simulink model "commit9"  (R2022a)
settings: Solver=VariableStepAuto  StartTime=0.0  StopTime=50  RelTol=1e-3
InitFcn:
  | uav_param, LQR_maker
undefined symbols (not defined in the file or in its folder): auto_LQR, Continuous, drawQuad, ff_splitter1, ff_splitter2, gr_eff, intrcptr_traj3, OL_LIN_maker, plotmavstatevariables, pos_comprtr, splitter1, Time, uav_P
libraries: ctrlSharedLib x1
settings Model: Creator=Abhi  LastModifiedBy=Abhi

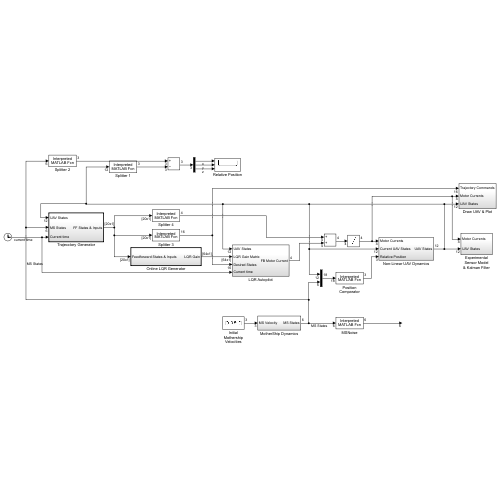
[thumbnail: Simulink's stored preview of the top-level diagram]
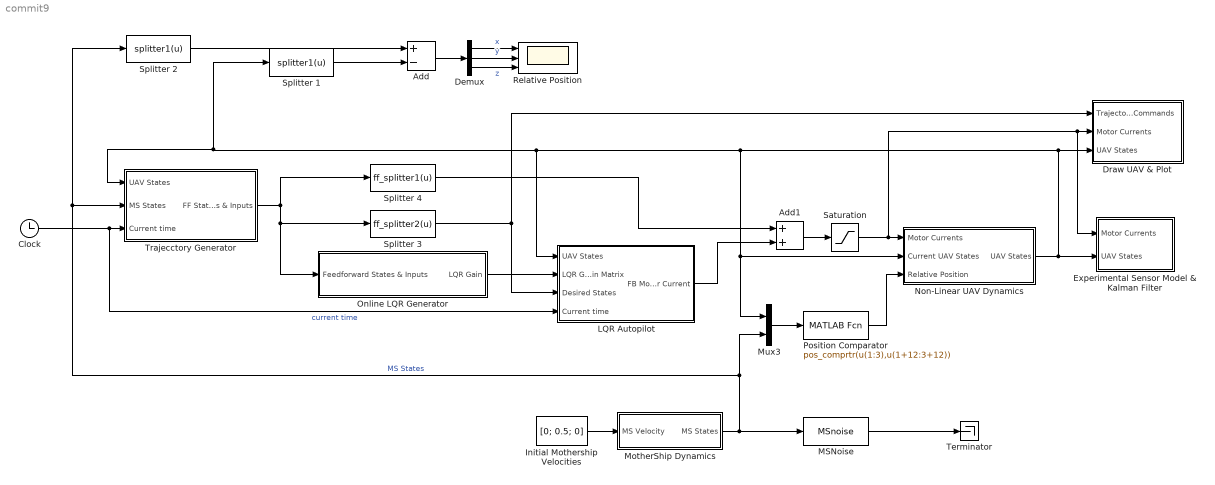
== system commit9 ==
  Add : Sum  Inputs=+-
  Add1 : Sum
  Clock : Clock
  Demux : Demux  Outputs=3
  Draw UAV & Plot : Subsystem
  Experimental Sensor Model & Kalman Filter : Subsystem
  Initial Mothership Velocities : Constant  Value=[0; 0.5; 0]
  LQR Autopilot : Subsystem
  MSNoise : MATLABFcn  MATLABFcn=MSnoise  OutputDimensions=6
  MotherShip Dynamics : Subsystem
  Mux3 : Mux  Inputs=2
  Non-Linear UAV Dynamics : Subsystem
  Online LQR Generator : Subsystem  TreatAsAtomicUnit=on  SystemSampleTime=1
  Position Comparator : MATLABFcn  MATLABFcn=pos_comprtr(u(1:3),u(1+12:3+12))
  Relative Position : Scope  NumInputPorts=3
  Saturation : Saturate  UpperLimit=4  LowerLimit=0  ZeroCross=off
  Splitter 1 : MATLABFcn  MATLABFcn=splitter1(u)
  Splitter 2 : MATLABFcn  MATLABFcn=splitter1(u)
  Splitter 3 : MATLABFcn  MATLABFcn=ff_splitter2(u)
  Splitter 4 : MATLABFcn  MATLABFcn=ff_splitter1(u)
  Terminator : Terminator
  Trajecctory Generator : Subsystem  TreatAsAtomicUnit=on  SystemSampleTime=2.5
  wires:
  Initial Mothership Velocities/1 -> MotherShip Dynamics/1(MS Velocity)
  MSNoise/1 -> Terminator/1
  Mux3/1 -> Position Comparator/1
  Position Comparator/1 -> Non-Linear UAV Dynamics/3(Relative Position)
  Add1/1 -> Saturation/1
  Splitter 4/1 -> Add1/1
  Splitter 3/1 -> LQR Autopilot/3(Desired States), Draw UAV & Plot/1(Trajectory Commands)
  Saturation/1 -> Non-Linear UAV Dynamics/1(Motor Currents), Experimental Sensor Model & Kalman Filter/1(Motor Currents), Draw UAV & Plot/2(Motor Currents)
  Trajecctory Generator/1(FF States & Inputs) -> Online LQR Generator/1(Feedforward States & Inputs), Splitter 3/1, Splitter 4/1
  Non-Linear UAV Dynamics/1(UAV States) -> Experimental Sensor Model & Kalman Filter/2(UAV States), Splitter 1/1, Trajecctory Generator/1(UAV States), LQR Autopilot/1(UAV States), Mux3/1, Non-Linear UAV Dynamics/2(Current UAV States), Draw UAV & Plot/3(UAV States)
  Splitter 2/1 -> Add/1
  Clock/1 -> LQR Autopilot/4(Current time), Trajecctory Generator/3(Current time)  "current time"
  Online LQR Generator/1(LQR Gain) -> LQR Autopilot/2(LQR Gain Matrix)
  Splitter 1/1 -> Add/2
  LQR Autopilot/1(FB Motor Current) -> Add1/2
  MotherShip Dynamics/1(MS States) -> MSNoise/1, Splitter 2/1, Trajecctory Generator/2(MS States), Mux3/2  "MS States"
  Demux/1 -> Relative Position/1  "x"
  Demux/2 -> Relative Position/2  "y"
  Demux/3 -> Relative Position/3  "z"
  Add/1 -> Demux/1

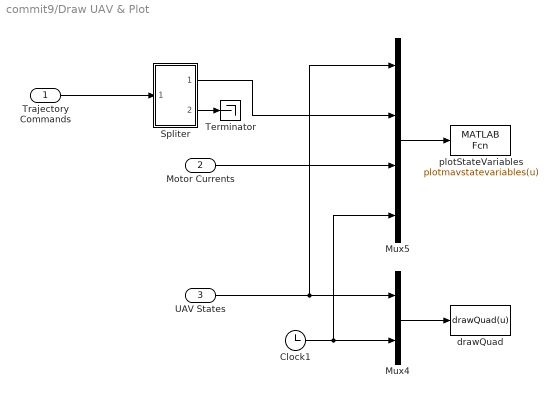
== system commit9/Draw UAV & Plot ==
  Trajectory Commands : Inport
  Motor Currents : Inport  Port=2
  UAV States : Inport  Port=3
  Clock1 : Clock
  Mux4 : Mux  Inputs=2
  Mux5 : Mux
  Spliter : Subsystem
  Terminator : Terminator
  drawQuad : MATLABFcn  MATLABFcn=drawQuad(u)  OutputDimensions=0  SampleTime=0.1
  plotStateVariables : MATLABFcn  MATLABFcn=plotmavstatevariables(u)  OutputDimensions=0  SampleTime=0.1
  wires:
  Mux4/1 -> drawQuad/1
  Mux5/1 -> plotStateVariables/1
  UAV States/1 -> Mux4/1, Mux5/1
  Clock1/1 -> Mux4/2, Mux5/4
  Motor Currents/1 -> Mux5/3
  Trajectory Commands/1 -> Spliter/1(Calculated Trajectory Commands)
  Spliter/1(UAV States) -> Mux5/2
  Spliter/2(Out2) -> Terminator/1

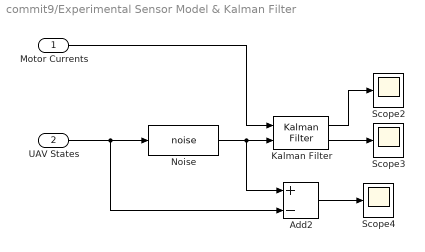
== system commit9/Experimental Sensor Model & Kalman Filter ==
  Motor Currents : Inport
  UAV States : Inport  Port=2
  Add2 : Sum  Inputs=+-
  Kalman Filter : ctrlSharedLib/Kalman Filter  TimeDomain=Continuous-Time  UseCurrentEstimator=on  ModelSource=Individual A, B, C, D matrices  ModelSourceVariable=ss(0.95,1,1,0,1)  A=uav_P.A  B=uav_P.B  C=uav_P.C  D=uav_P.D  NumberOfStates=1  NumberOfInputs=1  NumberOfOutputs=1  InitialEstimateSource=Dialog  X0=uav_P.INIT  P0=10  UseK=off  UseGH=off  NumberOfProcessNoiseInputs=1  G=1  TimeInvariantG=on  H=0  TimeInvariantH=on  Q=uav_P.QQ  TimeInvariantQ=on  R=uav_P.RR  TimeInvariantR=on  N=0  TimeInvariantN=on  AddInputPort=on  AddEnablePort=off  OutputEstimatedY=on  OutputP=off  Ts=-1
  Noise : MATLABFcn  MATLABFcn=noise  OutputDimensions=12
  Scope2 : Scope
  Scope3 : Scope
  Scope4 : Scope
  wires:
  UAV States/1 -> Noise/1, Add2/2
  Noise/1 -> Kalman Filter/2, Add2/1
  Kalman Filter/2 -> Scope3/1
  Add2/1 -> Scope4/1
  Kalman Filter/1 -> Scope2/1
  Motor Currents/1 -> Kalman Filter/1

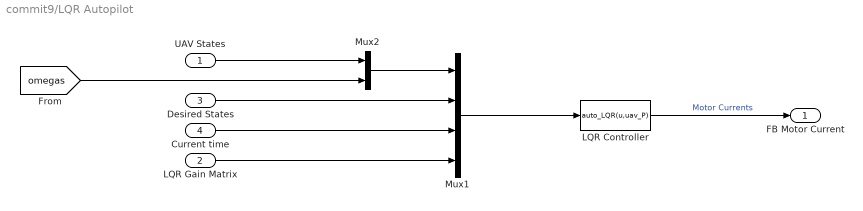
== system commit9/LQR Autopilot ==
  UAV States : Inport
  LQR Gain Matrix : Inport  Port=2
  Desired States : Inport  Port=3
  Current time : Inport  Port=4
  LQR Controller : MATLABFcn  MATLABFcn=auto_LQR(u,uav_P)
  Mux1 : Mux
  Mux2 : Mux  Inputs=2
  FB Motor Current : Outport
  wires:
  Desired States/1 -> Mux1/2
  LQR Controller/1 -> FB Motor Current/1  "Motor Currents"
  [omegas] -> Mux2/2
  Mux2/1 -> Mux1/1
  UAV States/1 -> Mux2/1
  Current time/1 -> Mux1/3
  Mux1/1 -> LQR Controller/1
  LQR Gain Matrix/1 -> Mux1/4

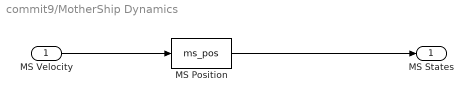
== system commit9/MotherShip Dynamics ==
  MS Velocity : Inport
  MS Position : S-Function  FunctionName=ms_pos  Parameters=x0_ms  SFunctionDeploymentMode=off  EnableBusSupport=off
  MS States : Outport
  wires:
  MS Velocity/1 -> MS Position/1
  MS Position/1 -> MS States/1

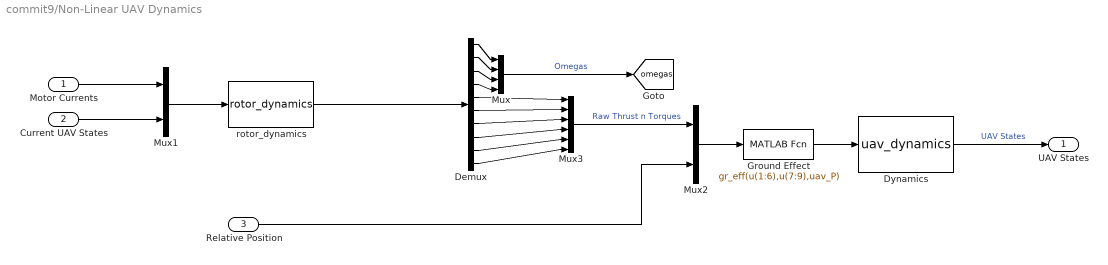
== system commit9/Non-Linear UAV Dynamics ==
  Motor Currents : Inport
  Current UAV States : Inport  Port=2
  Relative Position : Inport  Port=3
  Demux : Demux  Outputs=10
  Dynamics : S-Function  FunctionName=uav_dynamics  Parameters=uav_P  SFunctionDeploymentMode=off  EnableBusSupport=off
  Ground Effect : MATLABFcn  MATLABFcn=gr_eff(u(1:6),u(7:9),uav_P)
  Mux : Mux
  Mux1 : Mux  Inputs=2
  Mux2 : Mux  Inputs=2
  Mux3 : Mux  Inputs=6
  rotor_dynamics : S-Function  FunctionName=rotor_dynamics  Parameters=uav_P  SFunctionDeploymentMode=off  EnableBusSupport=off
  UAV States : Outport
  tag scope: omegas=global
  wires:
  Mux2/1 -> Ground Effect/1
  Dynamics/1 -> UAV States/1  "UAV States"
  Current UAV States/1 -> Mux1/2
  Relative Position/1 -> Mux2/2
  Motor Currents/1 -> Mux1/1
  Ground Effect/1 -> Dynamics/1
  Mux1/1 -> rotor_dynamics/1
  rotor_dynamics/1 -> Demux/1
  Demux/5 -> Mux3/1
  Demux/8 -> Mux3/4
  Demux/7 -> Mux3/3
  Demux/1 -> Mux/1
  Demux/3 -> Mux/3
  Demux/10 -> Mux3/6
  Demux/2 -> Mux/2
  Mux3/1 -> Mux2/1  "Raw Thrust n Torques"
  Mux/1 -> [omegas]  "Omegas"
  Demux/6 -> Mux3/2
  Demux/4 -> Mux/4
  Demux/9 -> Mux3/5

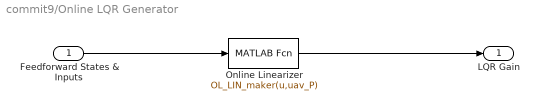
== system commit9/Online LQR Generator ==
  Feedforward States & Inputs : Inport
  Online Linearizer : MATLABFcn  MATLABFcn=OL_LIN_maker(u,uav_P)  OutputDimensions=[64,1]  Output1D=off
  LQR Gain : Outport
  wires:
  Feedforward States & Inputs/1 -> Online Linearizer/1
  Online Linearizer/1 -> LQR Gain/1

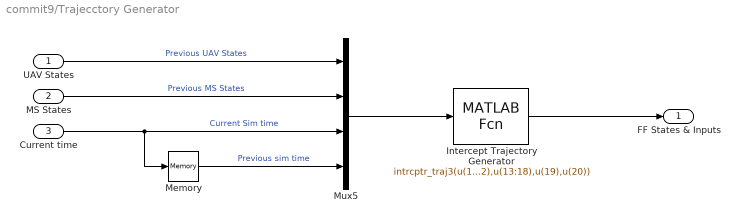
== system commit9/Trajecctory Generator ==
  UAV States : Inport
  MS States : Inport  Port=2
  Current time : Inport  Port=3
  Intercept Trajectory Generator : MATLABFcn  MATLABFcn=intrcptr_traj3(u(1:12),u(13:18),u(19),u(20))  OutputDimensions=[20,1]  Output1D=off
  Memory : Memory  InheritSampleTime=on
  Mux5 : Mux
  FF States & Inputs : Outport
  wires:
  Memory/1 -> Mux5/4  "Previous sim time"
  Current time/1 -> Mux5/3, Memory/1  "Current Sim time"
  Mux5/1 -> Intercept Trajectory Generator/1
  Intercept Trajectory Generator/1 -> FF States & Inputs/1
  UAV States/1 -> Mux5/1  "Previous UAV States"
  MS States/1 -> Mux5/2  "Previous MS States"

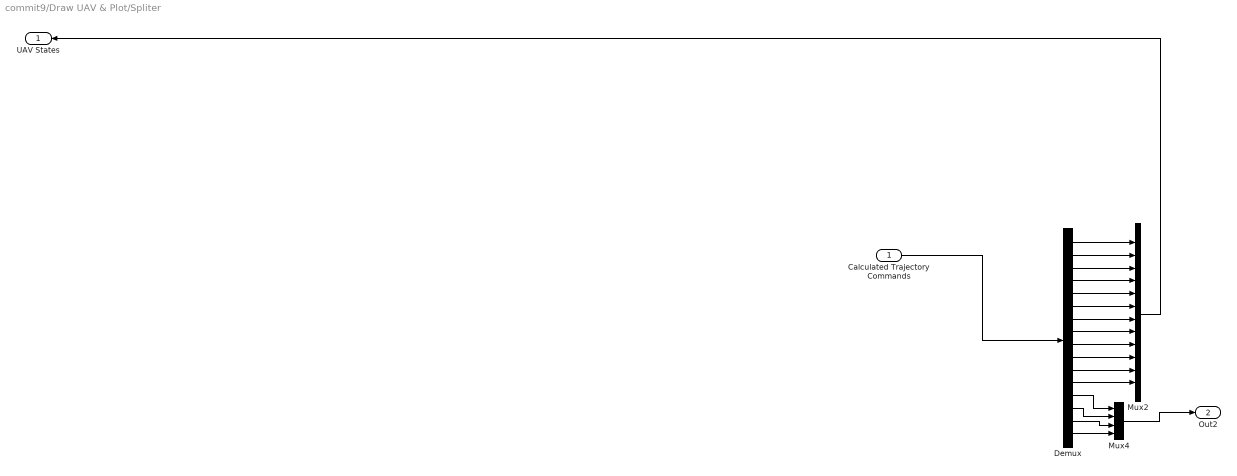
== system commit9/Draw UAV & Plot/Spliter ==
  Calculated Trajectory Commands : Inport
  Demux : Demux  Outputs=16
  Mux2 : Mux  Inputs=12
  Mux4 : Mux
  UAV States : Outport
  Out2 : Outport  Port=2
  wires:
  Demux/3 -> Mux2/3
  Demux/6 -> Mux2/6
  Demux/9 -> Mux2/9
  Demux/2 -> Mux2/2
  Demux/16 -> Mux4/4
  Demux/13 -> Mux4/1
  Demux/4 -> Mux2/4
  Demux/7 -> Mux2/7
  Mux2/1 -> UAV States/1
  Demux/10 -> Mux2/10
  Demux/11 -> Mux2/11
  Demux/8 -> Mux2/8
  Demux/15 -> Mux4/3
  Demux/1 -> Mux2/1
  Demux/12 -> Mux2/12
  Demux/14 -> Mux4/2
  Demux/5 -> Mux2/5
  Mux4/1 -> Out2/1
  Calculated Trajectory Commands/1 -> Demux/1
